simulink model "Simulink2"  (R2016b)
settings: Solver=VariableStepAuto  StartTime=0.0  StopTime=10.0  RelTol=1e-3
settings Model: Creator=ASUS  LastModifiedBy=ASUS

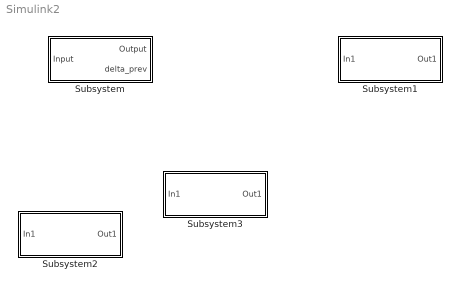
== system Simulink2 ==
  Subsystem : Subsystem
  Subsystem1 : Subsystem
  Subsystem2 : Subsystem
  Subsystem3 : Subsystem

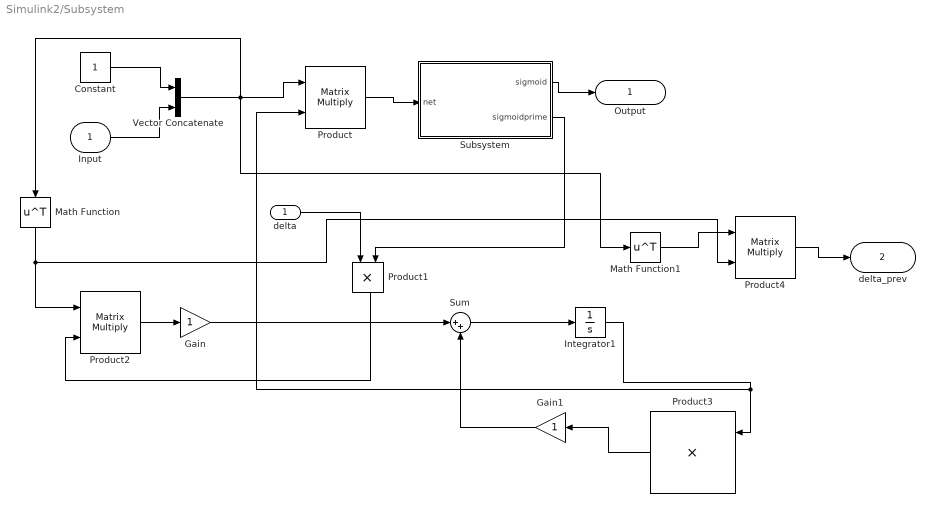
== system Simulink2/Subsystem ==
  "Input " : Inport
  Constant : Constant
  Gain : Gain
  Gain1 : Gain
  Integrator1 : Integrator
  Math Function : Math  Operator=transpose  SaturateOnIntegerOverflow=on
  Math Function1 : Math  Operator=transpose  SaturateOnIntegerOverflow=on
  Product : Product  Multiplication=Matrix(*)
  Product1 : Product
  Product2 : Product  Multiplication=Matrix(*)
  Product3 : Product
  Product4 : Product  Multiplication=Matrix(*)
  Subsystem : Subsystem
  Sum : Sum  Inputs=|++
  Vector Concatenate : Concatenate
  delta : InportShadow
  "Output " : Outport
  "delta_prev " : Outport  Port=2
  wires:
  "Input "/1 -> Vector Concatenate/2
  Constant/1 -> Vector Concatenate/1
  Vector Concatenate/1 -> Math Function1/1, Math Function/1, Product/1
  Product/1 -> Subsystem/1(net)
  Subsystem/2("sigmoidprime ") -> Product1/2
  delta/1 -> Product1/1
  Math Function/1 -> Product4/2, Product2/1
  Product1/1 -> Product2/2
  Product2/1 -> Gain/1
  Gain/1 -> Sum/1
  Sum/1 -> Integrator1/1
  Product3/1 -> Gain1/1
  Gain1/1 -> Sum/2
  Subsystem/1(sigmoid) -> "Output "/1
  Integrator1/1 -> Product3/1, Product/2
  Math Function1/1 -> Product4/1
  Product4/1 -> "delta_prev "/1

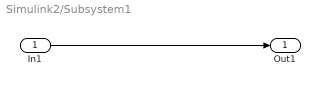
== system Simulink2/Subsystem1 ==
  In1 : Inport
  Out1 : Outport
  wires:
  In1/1 -> Out1/1

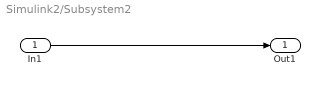
== system Simulink2/Subsystem2 ==
  In1 : Inport
  Out1 : Outport
  wires:
  In1/1 -> Out1/1

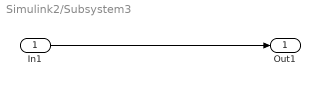
== system Simulink2/Subsystem3 ==
  In1 : Inport
  Out1 : Outport
  wires:
  In1/1 -> Out1/1

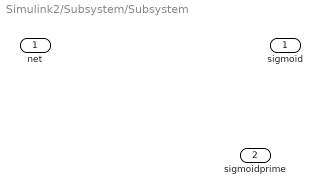
== system Simulink2/Subsystem/Subsystem ==
  net : Inport
  sigmoid : Outport
  "sigmoidprime " : Outport  Port=2
